simulink model "robot"  (R2025b)
settings: Solver=VariableStepAuto  StartTime=0.0  StopTime=10.0  RelTol=1e-3
settings Model: Creator=simoa  LastModifiedBy=simoa

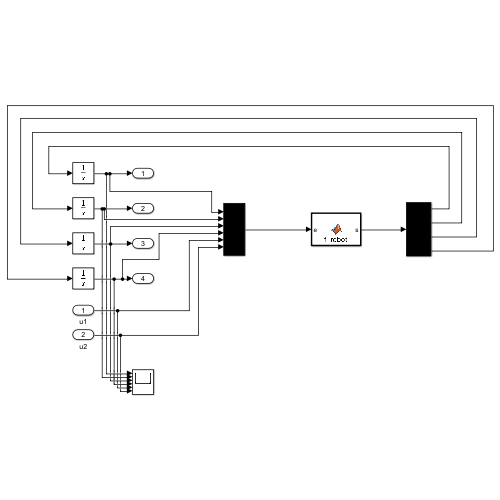
[thumbnail: Simulink's stored preview of the top-level diagram]
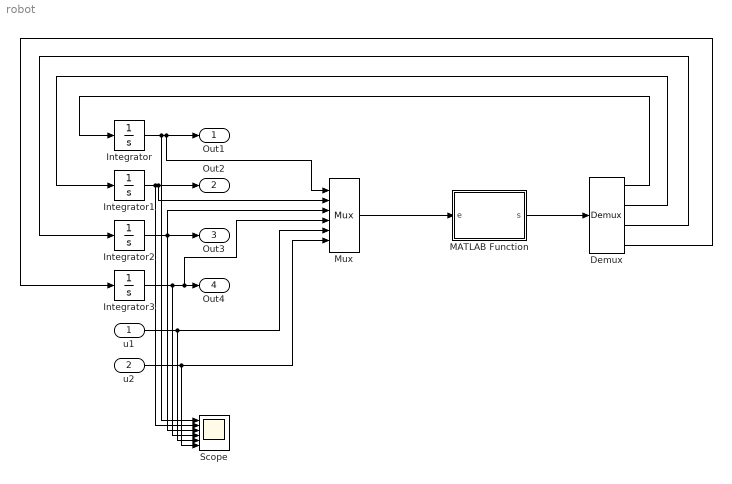
== system robot ==
  u1 : Inport
  u2 : Inport  Port=2
  Demux : Demux
  Integrator : Integrator  InitialCondition=0.01
  Integrator1 : Integrator
  Integrator2 : Integrator
  Integrator3 : Integrator
  MATLAB Function : MATLAB Function  TreatAsAtomicUnit=on
  Mux : Mux  Inputs=6
  Scope : Scope  NumInputPorts=6
  Out1 : Outport
  Out2 : Outport  Port=2
  Out3 : Outport  Port=3
  Out4 : Outport  Port=4
  wires:
  Mux/1 -> MATLAB Function/1(e)
  MATLAB Function/1(s) -> Demux/1
  Integrator/1 -> Scope/1, Mux/1, Out1/1
  Integrator1/1 -> Mux/2, Out2/1, Scope/2
  Integrator2/1 -> Scope/3, Mux/3, Out3/1
  Integrator3/1 -> Scope/4, Mux/4, Out4/1
  u1/1 -> Scope/5, Mux/5
  u2/1 -> Scope/6, Mux/6
  Demux/1 -> Integrator/1
  Demux/3 -> Integrator2/1
  Demux/4 -> Integrator3/1
  Demux/2 -> Integrator1/1

== matlab function robot/MATLAB Function ==
  data: e input; s output
function s = f_robot(e)
    % 1. System Parameters
    m = 1;      % Mass of the robot load
    g = 9.8;    % Gravity

    % 2. Map the Input Vector 'e'
    % The block receives 6 signals bundled together: 4 current states + 2 control inputs
    x1 = e(1);  % Radial position (r)
    x2 = e(2);  % Radial velocity (r_dot)
    x3 = e(3);  % Angular position (theta)
    x4 = e(4);  % Angular velocity (theta_dot)
    u1 = e(5);  % Control Force (F)
    u2 = e(6);  % Control Torque (T)

    % 3. Physics Equations (How the states change over time)
    dx1 = x2;
    dx2 = x1*x4^2 - g*sin(x3) + u1/m;
    dx3 = x4;
    dx4 = (-2*x1*x2*x4 - g*x1*cos(x3) + u2/m) / (x1^2);

    % 4. Output the changes
    s = [dx1; dx2; dx3; dx4];
end
